simulink model "model"  (R2020b)
settings: Solver=VariableStepAuto  StartTime=0.0  StopTime=inf  RelTol=1e-3
settings Model: Creator=Pavan  LastModifiedBy=Pavan

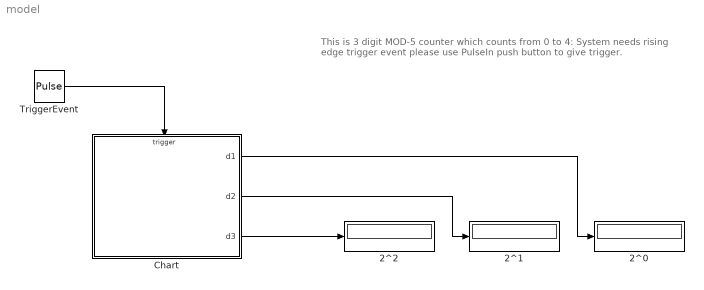
== system model ==
  note: This is 3 digit MOD-5 counter which counts from 0 to 4:
      |
      | System needs rising edge trigger event please use PulseIn push button to give trigger.
  2^0 : Display
  2^1 : Display
  2^2 : Display
  Chart : Stateflow chart  TreatAsAtomicUnit=on
  TriggerEvent : DiscretePulseGenerator  PulseType=Time based  Period=22000  PulseWidth=5
  wires:
  TriggerEvent/1 -> Chart/Trigger
  Chart/3(d3) -> 2^2/1
  Chart/2(d2) -> 2^1/1
  Chart/1(d1) -> 2^0/1

== stateflow chart model/Chart ==
  state Counter
    state FirstDigit [parallel]
      settings: executionOrder=1
      state initial
        en:d1=0;
        en:reset=0;
      state Zero
        en:d1=0;
      state One
        en:d1=1;
      initial -> Counter.FirstDigit.One : pulseIn
      (junction 45) -> initial [order 2] : [reset==1]
      Counter.FirstDigit.Zero -> (junction 45) : pulseIn
      (junction 45) -> Counter.FirstDigit.One [order 1] : [reset==0]
      (default) -> Counter.FirstDigit.Zero
      Counter.FirstDigit.One -> Counter.FirstDigit.Zero : pulseIn/{inc1;}
    state SecondDigit [parallel]
      settings: executionOrder=2
      state Zero
        en:d2=0;
      state One
        en:d2=1;
      (default) -> Counter.SecondDigit.Zero
      Counter.SecondDigit.Zero -> Counter.SecondDigit.One : inc1
      Counter.SecondDigit.One -> Counter.SecondDigit.Zero : inc1/{inc2;}
    state ThirdDigit [parallel]
      settings: executionOrder=3
      state Zero
        en:
        d3=0;
      state One
        en:d3=1;
        en:reset =1;
      Counter.ThirdDigit.Zero -> Counter.ThirdDigit.One : inc2
      (default) -> Counter.ThirdDigit.Zero
      Counter.ThirdDigit.One -> Counter.ThirdDigit.Zero : [reset ==0]
  (default) -> Counter
  data: d1 output; d2 output; d3 output; reset local =0
  events: pulseIn input RISING_EDGE_EVENT; inc1 local FUNCTION_CALL_EVENT; inc2 local FUNCTION_CALL_EVENT
